simulink model "Multi_drones_deri_compare"  (R2021a)
settings: Solver=ode4  StartTime=0.0  StopTime=50  FixedStep=0.005  RelTol=1e-3
(part 3 of 7)

== system Multi_drones_deri_compare/Controller 6/Controller/Attitude controller ==
  states_i : Inport
  atti_ref : Inport  Port=2
  u_nom_a : Inport  Port=3
  Angle controller : MATLAB Function  TreatAsAtomicUnit=on
  Angle error : MATLAB Function  TreatAsAtomicUnit=on
  Angle sliding variable : MATLAB Function  TreatAsAtomicUnit=on
  Attitude loop observer : Subsystem
      settings: PortSchema="{\"entries\":[{\"content\":{\"sides\":[{\"content\":{\"connectorIds\":[\"In1\",\"In2\",\"In3\"]},\"type\":\"ConnectorPlacement.EquallySpacedRectSide\",\"uuid\":\"edf82c9f-eb15-4775-9311-d50d92fa47fd\"},{\"content\":{\"connectorIds\":[\"Out1\",\"Out2\"],\"side\":\"RIGHT\"},\"type\":\"ConnectorPlacement.EquallySpacedRectSide\",\"uuid\":\"b90416f6-8117-4ec7-8f9a-c5fae9711eab\"},{\"content\":{\"connectorIds\":[\"In4\"],\"side\":\"TOP\"},\"type\":\"ConnectorPlacement.EquallySpacedRectSide\",\"uuid\":\"e7e2e1a9-76d3-420a-917d-b73182cbe298\"}]},\"type\":\"ConnectorPlacement.EquallySpacedConnector\",\"uuid\":\"4fc8298e-c3da-4bdd-b1ba-c07bafbec956\"}],\"packageUris\":[\"http://schema.mathworks.com/mf0/Connector/R2020b\"],\"version\":\"1.0\"}"
  Scope : Scope
  Sliding mode differentiator : Subsystem
      settings: PortSchema="{\"entries\":[{\"content\":{\"sides\":[{\"content\":{\"connectorIds\":[\"In1\"]},\"type\":\"ConnectorPlacement.EquallySpacedRectSide\",\"uuid\":\"d0355641-aeac-4820-b7cd-f9621efbd127\"},{\"content\":{\"connectorIds\":[\"Out1\",\"Out2\"],\"side\":\"RIGHT\"},\"type\":\"ConnectorPlacement.EquallySpacedRectSide\",\"uuid\":\"185ec072-6206-4946-bebc-a6564ad10b6f\"},{\"content\":{\"connectorIds\":[\"Out3\"],\"side\":\"TOP\"},\"type\":\"ConnectorPlacement.EquallySpacedRectSide\",\"uuid\":\"43c1499b-0abd-4d60-8d0e-f99edfc99abb\"}]},\"type\":\"ConnectorPlacement.EquallySpacedConnector\",\"uuid\":\"7137f0d1-a693-433d-9f21-56f33280b1ef\"}],\"packageUris\":[\"http://schema.mathworks.com/mf0/Connector/R2020b\"],\"version\":\"1.0\"}"
  State selection : MATLAB Function  TreatAsAtomicUnit=on
  delta_v_a_6 : Scope
  delta_x_a_6 : Scope
  s_i_a_6 : Scope
  u_I_a : Outport
  w_hat_a : Outport  Port=2
  wires:
  Angle controller/1(u_i_a) -> Scope/1, u_I_a/1
  Angle sliding variable/1(s_i_a) -> s_i_a_6/1, Angle controller/2(s_i_a)
  atti_ref/1 -> Sliding mode differentiator/1(Reference)
  states_i/1 -> State selection/1(states_i), Attitude loop observer/1(states_i)
  State selection/1(x_i_a) -> Attitude loop observer/2(x_i_a), Angle error/1(x_i_a)
  State selection/2(v_i_a) -> Attitude loop observer/3(v_i_a), Angle error/2(v_i_a)
  Sliding mode differentiator/3(ang_d) -> Angle error/3(ang_d)
  Angle error/1(delta_x_a) -> delta_x_a_6/1, Angle sliding variable/1(delta_x_a), Angle controller/3(delta_x_a)
  Angle error/2(delta_v_a) -> delta_v_a_6/1, Angle controller/4(delta_v_a), Angle sliding variable/2(delta_v_a)
  Attitude loop observer/2(w_hat_a) -> Angle controller/1(w_hat_a)
  Sliding mode differentiator/2(ang_d_ddot) -> Angle controller/5(ang_d_ddot)
  u_nom_a/1 -> Attitude loop observer/4(u_nom_a)
  Sliding mode differentiator/1(ang_d_dot) -> Angle error/4(ang_d_dot)
  Attitude loop observer/1(w_hat_a_actual) -> w_hat_a/1

== system Multi_drones_deri_compare/Controller 6/Controller/Position controller1 ==
  states_i : Inport
  ref_x_p : Inport  Port=2
  u_nom_p : Inport  Port=3
  Constant : Constant  Value=[0;0;0]  VectorParams1D=off
  Error calculation : MATLAB Function  TreatAsAtomicUnit=on
  Position loop observer : Subsystem  mask{InitialCondition=[0;-1;0]}
      mask prompts: InitialCondition "Simulink:blkprm_prompts:IntegratorInitCond"
      settings: PortSchema="{\"entries\":[{\"content\":{\"sides\":[{\"content\":{\"connectorIds\":[\"In1\",\"In2\",\"In3\"]},\"type\":\"ConnectorPlacement.EquallySpacedRectSide\",\"uuid\":\"edf82c9f-eb15-4775-9311-d50d92fa47fd\"},{\"content\":{\"connectorIds\":[\"Out1\",\"Out2\"],\"side\":\"RIGHT\"},\"type\":\"ConnectorPlacement.EquallySpacedRectSide\",\"uuid\":\"b90416f6-8117-4ec7-8f9a-c5fae9711eab\"},{\"content\":{\"connectorIds\":[\"In4\"],\"side\":\"TOP\"},\"type\":\"ConnectorPlacement.EquallySpacedRectSide\",\"uuid\":\"e7e2e1a9-76d3-420a-917d-b73182cbe298\"}]},\"type\":\"ConnectorPlacement.EquallySpacedConnector\",\"uuid\":\"4fc8298e-c3da-4bdd-b1ba-c07bafbec956\"}],\"packageUris\":[\"http://schema.mathworks.com/mf0/Connector/R2020b\"],\"version\":\"1.0\"}"
      mask TypeOptions InitialCondition: x_int/InitialCondition
      mask DialogControl InitialCondition Prompt: Initial condition:
  Reference selection (Low) : MATLAB Function  TreatAsAtomicUnit=on
  State selection : MATLAB Function  TreatAsAtomicUnit=on
  Virtual position controller : MATLAB Function  TreatAsAtomicUnit=on
  delta_v_p_6 : Scope
  delta_x_p_6 : Scope
  s_i_p_6 : Scope
  u_i : Scope
  u_i_p : Outport
  w_hat_p : Outport  Port=2
  wires:
  states_i/1 -> Position loop observer/1(states_i), State selection/1(states_i)
  ref_x_p/1 -> Reference selection (Low)/1(ref_x_p)
  Reference selection (Low)/1(x_i_p_d) -> Error calculation/4(x_i_p_d)
  Reference selection (Low)/2(v_i_p_d) -> Error calculation/5(v_i_p_d)
  State selection/2(v_i_p) -> Position loop observer/3(v_i_p), Error calculation/2(v_i_p)
  State selection/1(x_i_p) -> Position loop observer/2(x_i_p), Error calculation/1(x_i_p)
  u_nom_p/1 -> Position loop observer/4(u_nom_p)
  Position loop observer/2(w_hat_p) -> Virtual position controller/1(w_hat_p)
  Reference selection (Low)/3(a_i_p_d) -> Virtual position controller/5(a_i_p_d)
  Constant/1 -> Error calculation/3(Phi_i)
  Error calculation/3(delta_v_p) -> delta_v_p_6/1, Virtual position controller/4(delta_v_p)
  Error calculation/2(delta_x_p) -> delta_x_p_6/1, Virtual position controller/3(delta_x_p)
  Error calculation/1(s_i_p) -> s_i_p_6/1, Virtual position controller/2(s_i_p)
  Virtual position controller/1(u_i_p) -> u_i_p/1, u_i/1
  Position loop observer/1(w_hat_p_actual) -> w_hat_p/1

== system Multi_drones_deri_compare/Controller 6/Controller/Reverse calculation ==
  psi_id : Inport
  u_ip : Inport  Port=2
  states_i : Inport  Port=3
  Reverse calculation : MATLAB Function  TreatAsAtomicUnit=on
  State selection : MATLAB Function  TreatAsAtomicUnit=on
  atti_ref : Outport
  T_i_d : Outport  Port=2
  wires:
  Reverse calculation/2(T_i_d) -> T_i_d/1
  Reverse calculation/1(atti_ref) -> atti_ref/1
  states_i/1 -> State selection/1(states_i)
  State selection/1(x_i_a) -> Reverse calculation/3(x_i_a)
  u_ip/1 -> Reverse calculation/2(u_i_p)
  psi_id/1 -> Reverse calculation/1(psi_i_d)

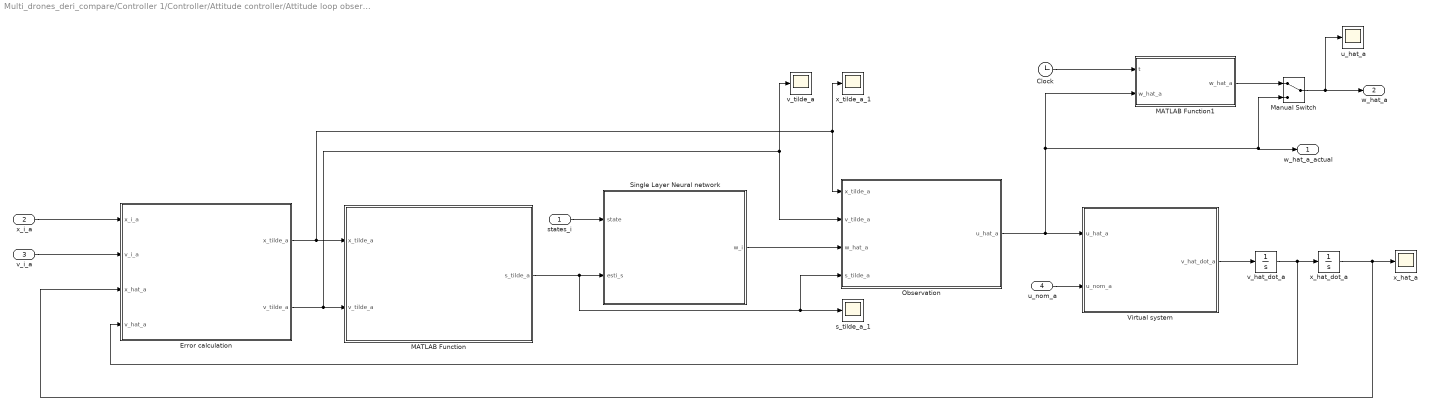
== system Multi_drones_deri_compare/Controller 1/Controller/Attitude controller/Attitude loop observer ==
  states_i : Inport
  x_i_a : Inport  Port=2
  v_i_a : Inport  Port=3
  u_nom_a : Inport  Port=4
  Clock : Clock
  Error calculation : MATLAB Function  TreatAsAtomicUnit=on
  MATLAB Function : MATLAB Function  TreatAsAtomicUnit=on
  MATLAB Function1 : MATLAB Function  TreatAsAtomicUnit=on
  Manual Switch : ManualSwitch
  Observation : MATLAB Function  TreatAsAtomicUnit=on
  Single Layer Neural network : Subsystem
  Virtual system : MATLAB Function  TreatAsAtomicUnit=on
  s_tilde_a_1 : Scope
  u_hat_a : Scope
  v_hat_dot_a : Integrator  InitialCondition=zeros(3,1)
  v_tilde_a : Scope
  x_hat_a : Scope
  x_hat_dot_a : Integrator  InitialCondition=zeros(3,1)
  x_tilde_a_1 : Scope
  w_hat_a_actual : Outport
  w_hat_a : Outport  Port=2
  wires:
  x_i_a/1 -> Error calculation/1(x_i_a)
  Error calculation/2(v_tilde_a) -> v_tilde_a/1, Observation/2(v_tilde_a), MATLAB Function/2(v_tilde_a)
  x_hat_dot_a/1 -> Error calculation/3(x_hat_a), x_hat_a/1
  v_hat_dot_a/1 -> Error calculation/4(v_hat_a), x_hat_dot_a/1
  MATLAB Function/1(s_tilde_a) -> Single Layer Neural network/2(esti_s), Observation/4(s_tilde_a), s_tilde_a_1/1
  Observation/1(u_hat_a) -> Manual Switch/2, w_hat_a_actual/1, MATLAB Function1/2("w_hat_a "), Virtual system/1(u_hat_a)
  u_nom_a/1 -> Virtual system/2(u_nom_a)
  v_i_a/1 -> Error calculation/2(v_i_a)
  Virtual system/1(v_hat_dot_a) -> v_hat_dot_a/1
  Error calculation/1(x_tilde_a) -> x_tilde_a_1/1, Observation/1(x_tilde_a), MATLAB Function/1(x_tilde_a)
  Single Layer Neural network/1(w_i) -> Observation/3(w_hat_a)
  states_i/1 -> Single Layer Neural network/1(state)
  Clock/1 -> MATLAB Function1/1(t)
  MATLAB Function1/1(w_hat_a) -> Manual Switch/1
  Manual Switch/1 -> u_hat_a/1, w_hat_a/1

== system Multi_drones_deri_compare/Controller 1/Controller/Attitude controller/Sliding mode differentiator ==
  note: Update initial state
  Reference : Inport
  Clock : Clock
  Constant : Constant  Value=[0;0;0]
  First-order derivative : Subsystem
  Integrator : Integrator  Commented=on  InitialCondition=[0;0;0;0;0;0;0;0;0;0;0;0]  ContinuousStateAttributes='speed'
  MATLAB Function : MATLAB Function  Commented=on  TreatAsAtomicUnit=on
  Manual Switch : ManualSwitch
  Second-order derivative : Subsystem
  a_d_a : Scope
  satu_atti_ref_ddot : Saturate  UpperLimit=0.1  LowerLimit=-0.1
  satu_atti_ref_dot : Saturate  UpperLimit=0.2  LowerLimit=-0.2
  sliding mode differentiator : MATLAB Function  Commented=on  TreatAsAtomicUnit=on
  v_d_a : Scope
  x_d_a : Scope
  ang_d_dot : Outport
  ang_d_ddot : Outport  Port=2
  ang_d : Outport  Port=3
  wires:
  sliding mode differentiator/1(z_dot) -> Integrator/1
  Reference/1 -> sliding mode differentiator/2(x_d), x_d_a/1, First-order derivative/1(ang_d), ang_d/1
  Integrator/1 -> MATLAB Function/1(z), sliding mode differentiator/1(z)
  satu_atti_ref_ddot/1 -> Manual Switch/1, a_d_a/1
  Second-order derivative/1(ang_d_ddot) -> satu_atti_ref_ddot/1
  Manual Switch/1 -> ang_d_ddot/1
  Constant/1 -> Manual Switch/2
  satu_atti_ref_dot/1 -> v_d_a/1, ang_d_dot/1
  Clock/1 -> Second-order derivative/2(t), First-order derivative/2(t)
  First-order derivative/1(ang_d_dot) -> satu_atti_ref_dot/1, Second-order derivative/1(ang_d_dot)

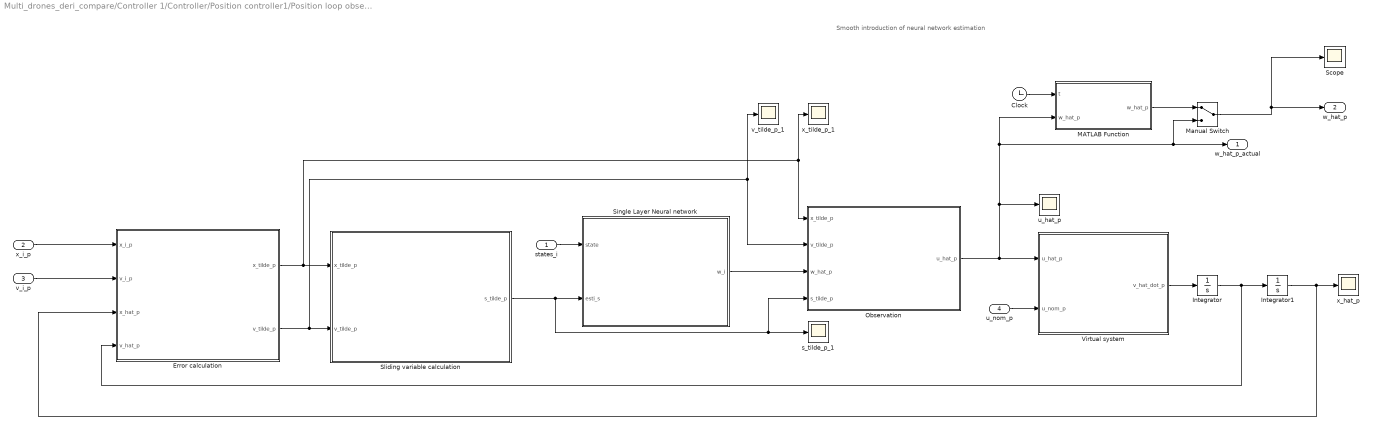
== system Multi_drones_deri_compare/Controller 1/Controller/Position controller1/Position loop observer ==
  note: Smooth introduction of neural network estimation
  states_i : Inport
  x_i_p : Inport  Port=2
  v_i_p : Inport  Port=3
  u_nom_p : Inport  Port=4
  Clock : Clock
  Error calculation : MATLAB Function  TreatAsAtomicUnit=on
  Integrator : Integrator  InitialCondition=[0;0;0]
  Integrator1 : Integrator  InitialCondition=InitialCondition
  MATLAB Function : MATLAB Function  TreatAsAtomicUnit=on
  Manual Switch : ManualSwitch
  Observation : MATLAB Function  TreatAsAtomicUnit=on
  Scope : Scope
  Single Layer Neural network : Subsystem
  Sliding variable calculation : MATLAB Function  TreatAsAtomicUnit=on
  Virtual system : MATLAB Function  TreatAsAtomicUnit=on
  s_tilde_p_1 : Scope
  u_hat_p : Scope
  v_tilde_p_1 : Scope
  x_hat_p : Scope
  x_tilde_p_1 : Scope
  w_hat_p_actual : Outport
  w_hat_p : Outport  Port=2
  wires:
  x_i_p/1 -> Error calculation/1(x_i_p)
  MATLAB Function/1(w_hat_p) -> Manual Switch/1
  Error calculation/2(v_tilde_p) -> v_tilde_p_1/1, Observation/2(v_tilde_p), Sliding variable calculation/2(v_tilde_p)
  Integrator1/1 -> Error calculation/3(x_hat_p), x_hat_p/1
  Integrator/1 -> Integrator1/1, Error calculation/4(v_hat_p)
  Sliding variable calculation/1(s_tilde_p) -> Single Layer Neural network/2(esti_s), Observation/4(s_tilde_p), s_tilde_p_1/1
  Observation/1(u_hat_p) -> w_hat_p_actual/1, Manual Switch/2, MATLAB Function/2("w_hat_p "), u_hat_p/1, Virtual system/1(u_hat_p)
  u_nom_p/1 -> Virtual system/2(u_nom_p)
  v_i_p/1 -> Error calculation/2(v_i_p)
  Virtual system/1(v_hat_dot_p) -> Integrator/1
  Error calculation/1(x_tilde_p) -> x_tilde_p_1/1, Observation/1(x_tilde_p), Sliding variable calculation/1(x_tilde_p)
  Single Layer Neural network/1(w_i) -> Observation/3(w_hat_p)
  states_i/1 -> Single Layer Neural network/1(state)
  Clock/1 -> MATLAB Function/1(t)
  Manual Switch/1 -> Scope/1, w_hat_p/1

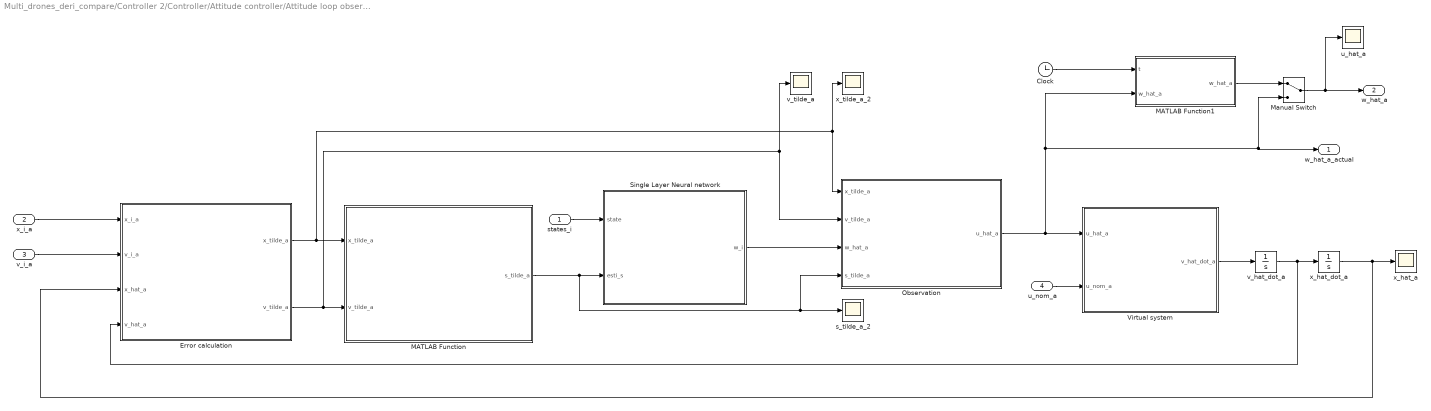
== system Multi_drones_deri_compare/Controller 2/Controller/Attitude controller/Attitude loop observer ==
  states_i : Inport
  x_i_a : Inport  Port=2
  v_i_a : Inport  Port=3
  u_nom_a : Inport  Port=4
  Clock : Clock
  Error calculation : MATLAB Function  TreatAsAtomicUnit=on
  MATLAB Function : MATLAB Function  TreatAsAtomicUnit=on
  MATLAB Function1 : MATLAB Function  TreatAsAtomicUnit=on
  Manual Switch : ManualSwitch
  Observation : MATLAB Function  TreatAsAtomicUnit=on
  Single Layer Neural network : Subsystem
  Virtual system : MATLAB Function  TreatAsAtomicUnit=on
  s_tilde_a_2 : Scope
  u_hat_a : Scope
  v_hat_dot_a : Integrator  InitialCondition=zeros(3,1)
  v_tilde_a : Scope
  x_hat_a : Scope
  x_hat_dot_a : Integrator  InitialCondition=zeros(3,1)
  x_tilde_a_2 : Scope
  w_hat_a_actual : Outport
  w_hat_a : Outport  Port=2
  wires:
  x_i_a/1 -> Error calculation/1(x_i_a)
  Error calculation/2(v_tilde_a) -> v_tilde_a/1, Observation/2(v_tilde_a), MATLAB Function/2(v_tilde_a)
  x_hat_dot_a/1 -> Error calculation/3(x_hat_a), x_hat_a/1
  v_hat_dot_a/1 -> Error calculation/4(v_hat_a), x_hat_dot_a/1
  MATLAB Function/1(s_tilde_a) -> Single Layer Neural network/2(esti_s), Observation/4(s_tilde_a), s_tilde_a_2/1
  Observation/1(u_hat_a) -> Manual Switch/2, w_hat_a_actual/1, MATLAB Function1/2("w_hat_a "), Virtual system/1(u_hat_a)
  u_nom_a/1 -> Virtual system/2(u_nom_a)
  v_i_a/1 -> Error calculation/2(v_i_a)
  Virtual system/1(v_hat_dot_a) -> v_hat_dot_a/1
  Error calculation/1(x_tilde_a) -> x_tilde_a_2/1, Observation/1(x_tilde_a), MATLAB Function/1(x_tilde_a)
  Single Layer Neural network/1(w_i) -> Observation/3(w_hat_a)
  states_i/1 -> Single Layer Neural network/1(state)
  Clock/1 -> MATLAB Function1/1(t)
  MATLAB Function1/1(w_hat_a) -> Manual Switch/1
  Manual Switch/1 -> u_hat_a/1, w_hat_a/1

== system Multi_drones_deri_compare/Controller 2/Controller/Attitude controller/Sliding mode differentiator ==
  note: Update initial state
  Reference : Inport
  Clock : Clock
  Constant : Constant  Value=[0;0;0]
  First-order derivative : Subsystem
  Integrator : Integrator  Commented=on  InitialCondition=[0;0;0;0;0;0;0;0;0;0;0;0]  ContinuousStateAttributes='speed'
  MATLAB Function : MATLAB Function  Commented=on  TreatAsAtomicUnit=on
  Manual Switch : ManualSwitch
  Second-order derivative : Subsystem
  a_d_a : Scope
  satu_atti_ref_ddot : Saturate  UpperLimit=0.2  LowerLimit=-0.2
  satu_atti_ref_dot : Saturate  UpperLimit=0.2  LowerLimit=-0.2
  sliding mode differentiator : MATLAB Function  Commented=on  TreatAsAtomicUnit=on
  v_d_a : Scope
  x_d_a : Scope
  ang_d_dot : Outport
  ang_d_ddot : Outport  Port=2
  ang_d : Outport  Port=3
  wires:
  sliding mode differentiator/1(z_dot) -> Integrator/1
  Reference/1 -> sliding mode differentiator/2(x_d), x_d_a/1, First-order derivative/1(ang_d), ang_d/1
  Integrator/1 -> MATLAB Function/1(z), sliding mode differentiator/1(z)
  satu_atti_ref_ddot/1 -> Manual Switch/1, a_d_a/1
  Second-order derivative/1(ang_d_ddot) -> satu_atti_ref_ddot/1
  Manual Switch/1 -> ang_d_ddot/1
  Constant/1 -> Manual Switch/2
  satu_atti_ref_dot/1 -> v_d_a/1, ang_d_dot/1
  Clock/1 -> Second-order derivative/2(t), First-order derivative/2(t)
  First-order derivative/1(ang_d_dot) -> satu_atti_ref_dot/1, Second-order derivative/1(ang_d_dot)

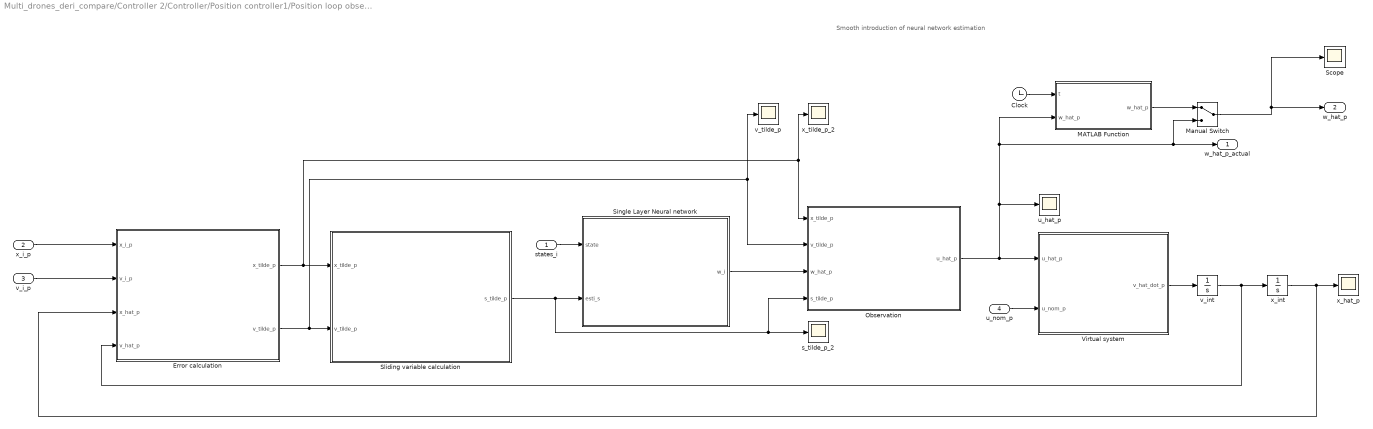
== system Multi_drones_deri_compare/Controller 2/Controller/Position controller1/Position loop observer ==
  note: Smooth introduction of neural network estimation
  states_i : Inport
  x_i_p : Inport  Port=2
  v_i_p : Inport  Port=3
  u_nom_p : Inport  Port=4
  Clock : Clock
  Error calculation : MATLAB Function  TreatAsAtomicUnit=on
  MATLAB Function : MATLAB Function  TreatAsAtomicUnit=on
  Manual Switch : ManualSwitch
  Observation : MATLAB Function  TreatAsAtomicUnit=on
  Scope : Scope
  Single Layer Neural network : Subsystem
  Sliding variable calculation : MATLAB Function  TreatAsAtomicUnit=on
  Virtual system : MATLAB Function  TreatAsAtomicUnit=on
  s_tilde_p_2 : Scope
  u_hat_p : Scope
  v_int : Integrator  InitialCondition=[0;0;0]
  v_tilde_p : Scope
  x_hat_p : Scope
  x_int : Integrator  InitialCondition=InitialCondition
  x_tilde_p_2 : Scope
  w_hat_p_actual : Outport
  w_hat_p : Outport  Port=2
  wires:
  x_i_p/1 -> Error calculation/1(x_i_p)
  MATLAB Function/1(w_hat_p) -> Manual Switch/1
  Error calculation/2(v_tilde_p) -> v_tilde_p/1, Observation/2(v_tilde_p), Sliding variable calculation/2(v_tilde_p)
  x_int/1 -> Error calculation/3(x_hat_p), x_hat_p/1
  v_int/1 -> x_int/1, Error calculation/4(v_hat_p)
  Sliding variable calculation/1(s_tilde_p) -> Single Layer Neural network/2(esti_s), Observation/4(s_tilde_p), s_tilde_p_2/1
  Observation/1(u_hat_p) -> w_hat_p_actual/1, Manual Switch/2, MATLAB Function/2("w_hat_p "), u_hat_p/1, Virtual system/1(u_hat_p)
  u_nom_p/1 -> Virtual system/2(u_nom_p)
  v_i_p/1 -> Error calculation/2(v_i_p)
  Virtual system/1(v_hat_dot_p) -> v_int/1
  Error calculation/1(x_tilde_p) -> x_tilde_p_2/1, Observation/1(x_tilde_p), Sliding variable calculation/1(x_tilde_p)
  Single Layer Neural network/1(w_i) -> Observation/3(w_hat_p)
  states_i/1 -> Single Layer Neural network/1(state)
  Clock/1 -> MATLAB Function/1(t)
  Manual Switch/1 -> Scope/1, w_hat_p/1

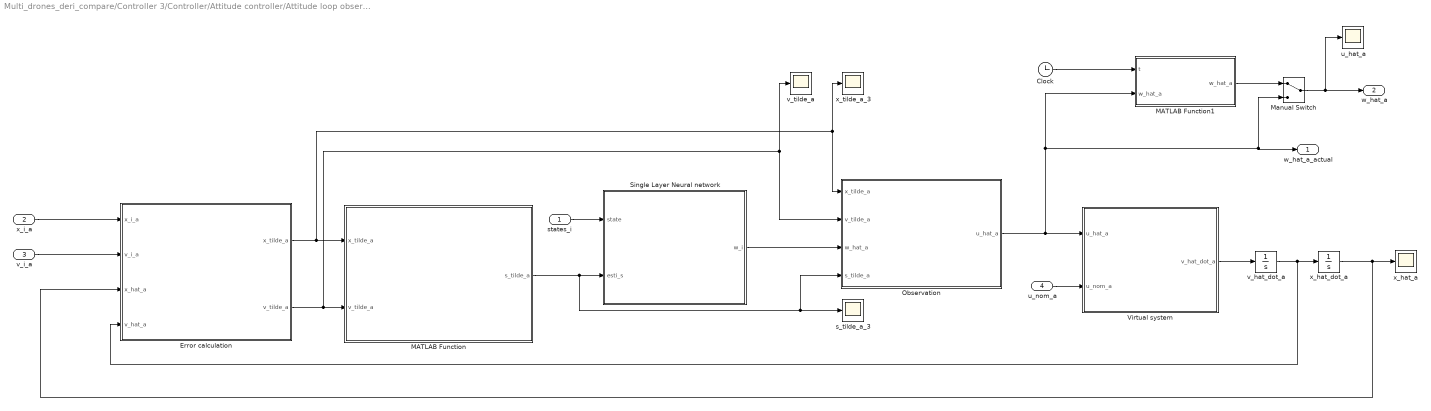
== system Multi_drones_deri_compare/Controller 3/Controller/Attitude controller/Attitude loop observer ==
  states_i : Inport
  x_i_a : Inport  Port=2
  v_i_a : Inport  Port=3
  u_nom_a : Inport  Port=4
  Clock : Clock
  Error calculation : MATLAB Function  TreatAsAtomicUnit=on
  MATLAB Function : MATLAB Function  TreatAsAtomicUnit=on
  MATLAB Function1 : MATLAB Function  TreatAsAtomicUnit=on
  Manual Switch : ManualSwitch
  Observation : MATLAB Function  TreatAsAtomicUnit=on
  Single Layer Neural network : Subsystem
  Virtual system : MATLAB Function  TreatAsAtomicUnit=on
  s_tilde_a_3 : Scope
  u_hat_a : Scope
  v_hat_dot_a : Integrator  InitialCondition=zeros(3,1)
  v_tilde_a : Scope
  x_hat_a : Scope
  x_hat_dot_a : Integrator  InitialCondition=zeros(3,1)
  x_tilde_a_3 : Scope
  w_hat_a_actual : Outport
  w_hat_a : Outport  Port=2
  wires:
  x_i_a/1 -> Error calculation/1(x_i_a)
  Error calculation/2(v_tilde_a) -> v_tilde_a/1, Observation/2(v_tilde_a), MATLAB Function/2(v_tilde_a)
  x_hat_dot_a/1 -> Error calculation/3(x_hat_a), x_hat_a/1
  v_hat_dot_a/1 -> Error calculation/4(v_hat_a), x_hat_dot_a/1
  MATLAB Function/1(s_tilde_a) -> Single Layer Neural network/2(esti_s), Observation/4(s_tilde_a), s_tilde_a_3/1
  Observation/1(u_hat_a) -> w_hat_a_actual/1, Manual Switch/2, MATLAB Function1/2("w_hat_a "), Virtual system/1(u_hat_a)
  u_nom_a/1 -> Virtual system/2(u_nom_a)
  v_i_a/1 -> Error calculation/2(v_i_a)
  Virtual system/1(v_hat_dot_a) -> v_hat_dot_a/1
  Error calculation/1(x_tilde_a) -> x_tilde_a_3/1, Observation/1(x_tilde_a), MATLAB Function/1(x_tilde_a)
  Single Layer Neural network/1(w_i) -> Observation/3(w_hat_a)
  states_i/1 -> Single Layer Neural network/1(state)
  Clock/1 -> MATLAB Function1/1(t)
  MATLAB Function1/1(w_hat_a) -> Manual Switch/1
  Manual Switch/1 -> u_hat_a/1, w_hat_a/1

== system Multi_drones_deri_compare/Controller 3/Controller/Attitude controller/Sliding mode differentiator ==
  note: Update initial state
  Reference : Inport
  Clock : Clock
  Constant : Constant  Value=[0;0;0]
  First-order derivative : Subsystem
  Integrator : Integrator  Commented=on  InitialCondition=[0;0;0;0;0;0;0;0;0;0;0;0]  ContinuousStateAttributes='speed'
  MATLAB Function : MATLAB Function  Commented=on  TreatAsAtomicUnit=on
  Manual Switch : ManualSwitch
  Second-order derivative : Subsystem
  a_d_a : Scope
  satu_atti_ref_ddot : Saturate  UpperLimit=0.2  LowerLimit=-0.2
  satu_atti_ref_dot : Saturate  UpperLimit=0.2  LowerLimit=-0.2
  sliding mode differentiator : MATLAB Function  Commented=on  TreatAsAtomicUnit=on
  v_d_a : Scope
  x_d_a : Scope
  ang_d_dot : Outport
  ang_d_ddot : Outport  Port=2
  ang_d : Outport  Port=3
  wires:
  sliding mode differentiator/1(z_dot) -> Integrator/1
  Reference/1 -> sliding mode differentiator/2(x_d), x_d_a/1, First-order derivative/1(ang_d), ang_d/1
  Integrator/1 -> MATLAB Function/1(z), sliding mode differentiator/1(z)
  satu_atti_ref_ddot/1 -> Manual Switch/1, a_d_a/1
  Second-order derivative/1(ang_d_ddot) -> satu_atti_ref_ddot/1
  Manual Switch/1 -> ang_d_ddot/1
  Constant/1 -> Manual Switch/2
  satu_atti_ref_dot/1 -> v_d_a/1, ang_d_dot/1
  Clock/1 -> Second-order derivative/2(t), First-order derivative/2(t)
  First-order derivative/1(ang_d_dot) -> satu_atti_ref_dot/1, Second-order derivative/1(ang_d_dot)

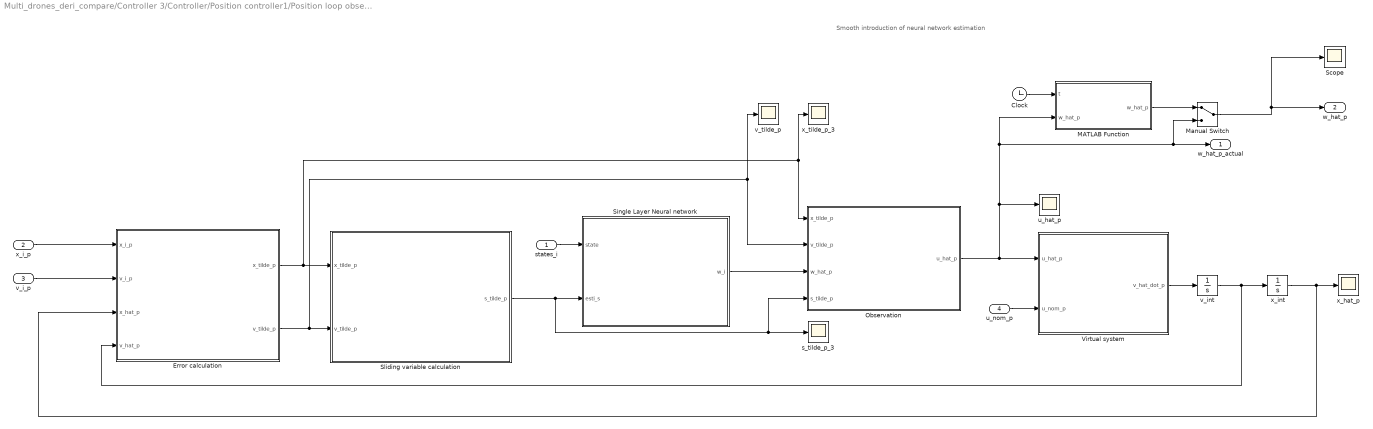
== system Multi_drones_deri_compare/Controller 3/Controller/Position controller1/Position loop observer ==
  note: Smooth introduction of neural network estimation
  states_i : Inport
  x_i_p : Inport  Port=2
  v_i_p : Inport  Port=3
  u_nom_p : Inport  Port=4
  Clock : Clock
  Error calculation : MATLAB Function  TreatAsAtomicUnit=on
  MATLAB Function : MATLAB Function  TreatAsAtomicUnit=on
  Manual Switch : ManualSwitch
  Observation : MATLAB Function  TreatAsAtomicUnit=on
  Scope : Scope
  Single Layer Neural network : Subsystem
  Sliding variable calculation : MATLAB Function  TreatAsAtomicUnit=on
  Virtual system : MATLAB Function  TreatAsAtomicUnit=on
  s_tilde_p_3 : Scope
  u_hat_p : Scope
  v_int : Integrator  InitialCondition=[0;0;0]
  v_tilde_p : Scope
  x_hat_p : Scope
  x_int : Integrator  InitialCondition=InitialCondition
  x_tilde_p_3 : Scope
  w_hat_p_actual : Outport
  w_hat_p : Outport  Port=2
  wires:
  x_i_p/1 -> Error calculation/1(x_i_p)
  MATLAB Function/1(w_hat_p) -> Manual Switch/1
  Error calculation/2(v_tilde_p) -> v_tilde_p/1, Observation/2(v_tilde_p), Sliding variable calculation/2(v_tilde_p)
  x_int/1 -> Error calculation/3(x_hat_p), x_hat_p/1
  v_int/1 -> x_int/1, Error calculation/4(v_hat_p)
  Sliding variable calculation/1(s_tilde_p) -> Single Layer Neural network/2(esti_s), Observation/4(s_tilde_p), s_tilde_p_3/1
  Observation/1(u_hat_p) -> w_hat_p_actual/1, Manual Switch/2, MATLAB Function/2("w_hat_p "), u_hat_p/1, Virtual system/1(u_hat_p)
  u_nom_p/1 -> Virtual system/2(u_nom_p)
  v_i_p/1 -> Error calculation/2(v_i_p)
  Virtual system/1(v_hat_dot_p) -> v_int/1
  Error calculation/1(x_tilde_p) -> x_tilde_p_3/1, Observation/1(x_tilde_p), Sliding variable calculation/1(x_tilde_p)
  Single Layer Neural network/1(w_i) -> Observation/3(w_hat_p)
  states_i/1 -> Single Layer Neural network/1(state)
  Clock/1 -> MATLAB Function/1(t)
  Manual Switch/1 -> Scope/1, w_hat_p/1

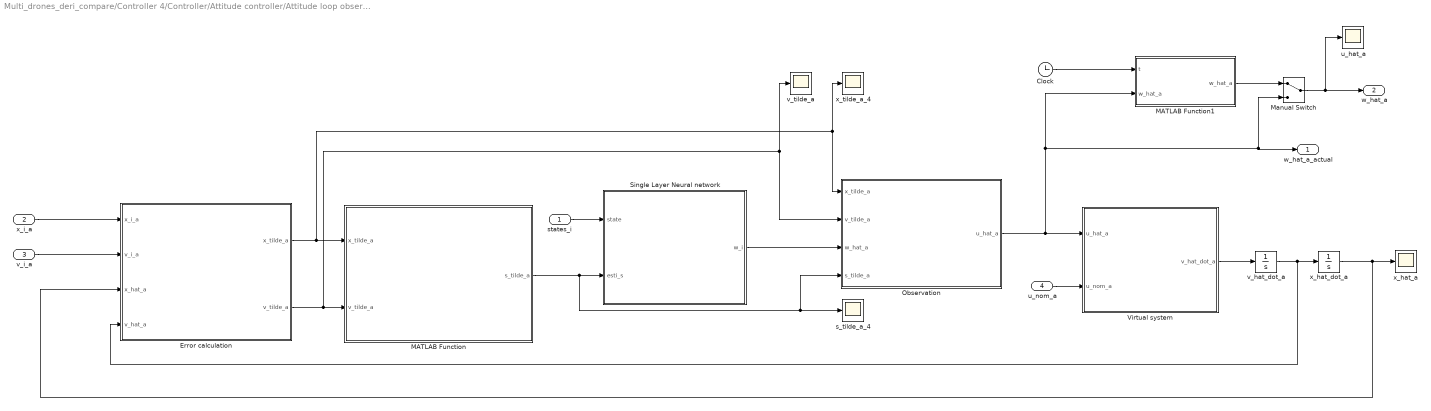
== system Multi_drones_deri_compare/Controller 4/Controller/Attitude controller/Attitude loop observer ==
  states_i : Inport
  x_i_a : Inport  Port=2
  v_i_a : Inport  Port=3
  u_nom_a : Inport  Port=4
  Clock : Clock
  Error calculation : MATLAB Function  TreatAsAtomicUnit=on
  MATLAB Function : MATLAB Function  TreatAsAtomicUnit=on
  MATLAB Function1 : MATLAB Function  TreatAsAtomicUnit=on
  Manual Switch : ManualSwitch
  Observation : MATLAB Function  TreatAsAtomicUnit=on
  Single Layer Neural network : Subsystem
  Virtual system : MATLAB Function  TreatAsAtomicUnit=on
  s_tilde_a_4 : Scope
  u_hat_a : Scope
  v_hat_dot_a : Integrator  InitialCondition=zeros(3,1)
  v_tilde_a : Scope
  x_hat_a : Scope
  x_hat_dot_a : Integrator  InitialCondition=zeros(3,1)
  x_tilde_a_4 : Scope
  w_hat_a_actual : Outport
  w_hat_a : Outport  Port=2
  wires:
  x_i_a/1 -> Error calculation/1(x_i_a)
  Error calculation/2(v_tilde_a) -> v_tilde_a/1, Observation/2(v_tilde_a), MATLAB Function/2(v_tilde_a)
  x_hat_dot_a/1 -> Error calculation/3(x_hat_a), x_hat_a/1
  v_hat_dot_a/1 -> Error calculation/4(v_hat_a), x_hat_dot_a/1
  MATLAB Function/1(s_tilde_a) -> Single Layer Neural network/2(esti_s), Observation/4(s_tilde_a), s_tilde_a_4/1
  Observation/1(u_hat_a) -> w_hat_a_actual/1, Manual Switch/2, MATLAB Function1/2("w_hat_a "), Virtual system/1(u_hat_a)
  u_nom_a/1 -> Virtual system/2(u_nom_a)
  v_i_a/1 -> Error calculation/2(v_i_a)
  Virtual system/1(v_hat_dot_a) -> v_hat_dot_a/1
  Error calculation/1(x_tilde_a) -> x_tilde_a_4/1, Observation/1(x_tilde_a), MATLAB Function/1(x_tilde_a)
  Single Layer Neural network/1(w_i) -> Observation/3(w_hat_a)
  states_i/1 -> Single Layer Neural network/1(state)
  Clock/1 -> MATLAB Function1/1(t)
  MATLAB Function1/1(w_hat_a) -> Manual Switch/1
  Manual Switch/1 -> u_hat_a/1, w_hat_a/1

== system Multi_drones_deri_compare/Controller 4/Controller/Attitude controller/Sliding mode differentiator ==
  note: Update initial state
  Reference : Inport
  Clock : Clock
  Constant : Constant  Value=[0;0;0]
  First-order derivative : Subsystem
  Integrator : Integrator  Commented=on  InitialCondition=[0;0;0;0;0;0;0;0;0;0;0;0]  ContinuousStateAttributes='speed'
  MATLAB Function : MATLAB Function  Commented=on  TreatAsAtomicUnit=on
  Manual Switch : ManualSwitch
  Second-order derivative : Subsystem
  a_d_a : Scope
  satu_atti_ref_ddot : Saturate  UpperLimit=0.2  LowerLimit=-0.2
  satu_atti_ref_dot : Saturate  UpperLimit=0.2  LowerLimit=-0.2
  sliding mode differentiator : MATLAB Function  Commented=on  TreatAsAtomicUnit=on
  v_d_a : Scope
  x_d_a : Scope
  ang_d_dot : Outport
  ang_d_ddot : Outport  Port=2
  ang_d : Outport  Port=3
  wires:
  sliding mode differentiator/1(z_dot) -> Integrator/1
  Reference/1 -> sliding mode differentiator/2(x_d), x_d_a/1, First-order derivative/1(ang_d), ang_d/1
  Integrator/1 -> MATLAB Function/1(z), sliding mode differentiator/1(z)
  satu_atti_ref_ddot/1 -> Manual Switch/1, a_d_a/1
  Second-order derivative/1(ang_d_ddot) -> satu_atti_ref_ddot/1
  Manual Switch/1 -> ang_d_ddot/1
  Constant/1 -> Manual Switch/2
  satu_atti_ref_dot/1 -> v_d_a/1, ang_d_dot/1
  Clock/1 -> Second-order derivative/2(t), First-order derivative/2(t)
  First-order derivative/1(ang_d_dot) -> satu_atti_ref_dot/1, Second-order derivative/1(ang_d_dot)

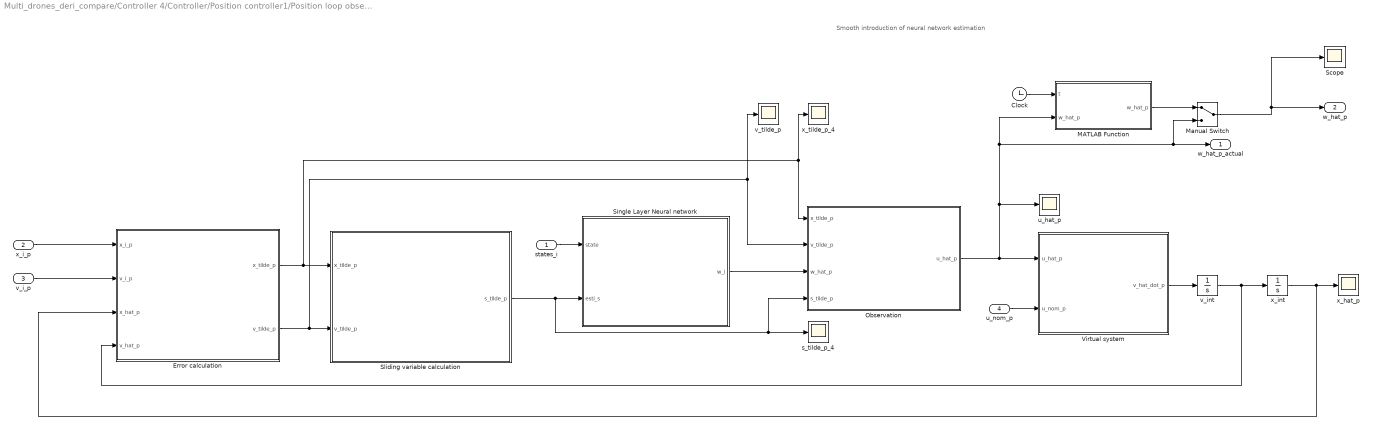
== system Multi_drones_deri_compare/Controller 4/Controller/Position controller1/Position loop observer ==
  note: Smooth introduction of neural network estimation
  states_i : Inport
  x_i_p : Inport  Port=2
  v_i_p : Inport  Port=3
  u_nom_p : Inport  Port=4
  Clock : Clock
  Error calculation : MATLAB Function  TreatAsAtomicUnit=on
  MATLAB Function : MATLAB Function  TreatAsAtomicUnit=on
  Manual Switch : ManualSwitch
  Observation : MATLAB Function  TreatAsAtomicUnit=on
  Scope : Scope
  Single Layer Neural network : Subsystem
  Sliding variable calculation : MATLAB Function  TreatAsAtomicUnit=on
  Virtual system : MATLAB Function  TreatAsAtomicUnit=on
  s_tilde_p_4 : Scope
  u_hat_p : Scope
  v_int : Integrator  InitialCondition=[0;0;0]
  v_tilde_p : Scope
  x_hat_p : Scope
  x_int : Integrator  InitialCondition=InitialCondition
  x_tilde_p_4 : Scope
  w_hat_p_actual : Outport
  w_hat_p : Outport  Port=2
  wires:
  x_i_p/1 -> Error calculation/1(x_i_p)
  MATLAB Function/1(w_hat_p) -> Manual Switch/1
  Error calculation/2(v_tilde_p) -> v_tilde_p/1, Observation/2(v_tilde_p), Sliding variable calculation/2(v_tilde_p)
  x_int/1 -> Error calculation/3(x_hat_p), x_hat_p/1
  v_int/1 -> x_int/1, Error calculation/4(v_hat_p)
  Sliding variable calculation/1(s_tilde_p) -> Single Layer Neural network/2(esti_s), Observation/4(s_tilde_p), s_tilde_p_4/1
  Observation/1(u_hat_p) -> w_hat_p_actual/1, Manual Switch/2, MATLAB Function/2("w_hat_p "), u_hat_p/1, Virtual system/1(u_hat_p)
  u_nom_p/1 -> Virtual system/2(u_nom_p)
  v_i_p/1 -> Error calculation/2(v_i_p)
  Virtual system/1(v_hat_dot_p) -> v_int/1
  Error calculation/1(x_tilde_p) -> x_tilde_p_4/1, Observation/1(x_tilde_p), Sliding variable calculation/1(x_tilde_p)
  Single Layer Neural network/1(w_i) -> Observation/3(w_hat_p)
  states_i/1 -> Single Layer Neural network/1(state)
  Clock/1 -> MATLAB Function/1(t)
  Manual Switch/1 -> Scope/1, w_hat_p/1

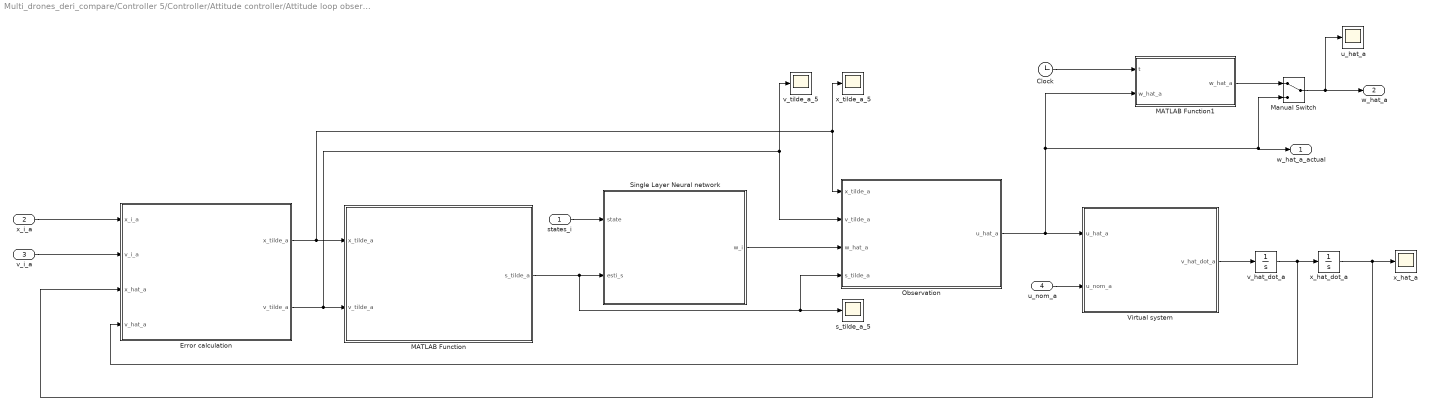
== system Multi_drones_deri_compare/Controller 5/Controller/Attitude controller/Attitude loop observer ==
  states_i : Inport
  x_i_a : Inport  Port=2
  v_i_a : Inport  Port=3
  u_nom_a : Inport  Port=4
  Clock : Clock
  Error calculation : MATLAB Function  TreatAsAtomicUnit=on
  MATLAB Function : MATLAB Function  TreatAsAtomicUnit=on
  MATLAB Function1 : MATLAB Function  TreatAsAtomicUnit=on
  Manual Switch : ManualSwitch
  Observation : MATLAB Function  TreatAsAtomicUnit=on
  Single Layer Neural network : Subsystem
  Virtual system : MATLAB Function  TreatAsAtomicUnit=on
  s_tilde_a_5 : Scope
  u_hat_a : Scope
  v_hat_dot_a : Integrator  InitialCondition=zeros(3,1)
  v_tilde_a_5 : Scope
  x_hat_a : Scope
  x_hat_dot_a : Integrator  InitialCondition=zeros(3,1)
  x_tilde_a_5 : Scope
  w_hat_a_actual : Outport
  w_hat_a : Outport  Port=2
  wires:
  x_i_a/1 -> Error calculation/1(x_i_a)
  Error calculation/2(v_tilde_a) -> v_tilde_a_5/1, Observation/2(v_tilde_a), MATLAB Function/2(v_tilde_a)
  x_hat_dot_a/1 -> Error calculation/3(x_hat_a), x_hat_a/1
  v_hat_dot_a/1 -> Error calculation/4(v_hat_a), x_hat_dot_a/1
  MATLAB Function/1(s_tilde_a) -> Single Layer Neural network/2(esti_s), Observation/4(s_tilde_a), s_tilde_a_5/1
  Observation/1(u_hat_a) -> Manual Switch/2, w_hat_a_actual/1, MATLAB Function1/2("w_hat_a "), Virtual system/1(u_hat_a)
  u_nom_a/1 -> Virtual system/2(u_nom_a)
  v_i_a/1 -> Error calculation/2(v_i_a)
  Virtual system/1(v_hat_dot_a) -> v_hat_dot_a/1
  Error calculation/1(x_tilde_a) -> x_tilde_a_5/1, Observation/1(x_tilde_a), MATLAB Function/1(x_tilde_a)
  Single Layer Neural network/1(w_i) -> Observation/3(w_hat_a)
  states_i/1 -> Single Layer Neural network/1(state)
  Clock/1 -> MATLAB Function1/1(t)
  MATLAB Function1/1(w_hat_a) -> Manual Switch/1
  Manual Switch/1 -> u_hat_a/1, w_hat_a/1

== system Multi_drones_deri_compare/Controller 5/Controller/Attitude controller/Sliding mode differentiator ==
  note: Update initial state
  Reference : Inport
  Clock : Clock
  Constant : Constant  Value=[0;0;0]
  First-order derivative : Subsystem
  Integrator : Integrator  Commented=on  InitialCondition=[0;0;0;0;0;0;0;0;0;0;0;0]  ContinuousStateAttributes='speed'
  MATLAB Function : MATLAB Function  Commented=on  TreatAsAtomicUnit=on
  Manual Switch : ManualSwitch
  Second-order derivative : Subsystem
  a_d_a : Scope
  satu_atti_ref_ddot : Saturate  UpperLimit=0.2  LowerLimit=-0.2
  satu_atti_ref_dot : Saturate  UpperLimit=0.2  LowerLimit=-0.2
  sliding mode differentiator : MATLAB Function  Commented=on  TreatAsAtomicUnit=on
  v_d_a : Scope
  x_d_a : Scope
  ang_d_dot : Outport
  ang_d_ddot : Outport  Port=2
  ang_d : Outport  Port=3
  wires:
  sliding mode differentiator/1(z_dot) -> Integrator/1
  Reference/1 -> sliding mode differentiator/2(x_d), x_d_a/1, First-order derivative/1(ang_d), ang_d/1
  Integrator/1 -> MATLAB Function/1(z), sliding mode differentiator/1(z)
  satu_atti_ref_ddot/1 -> Manual Switch/1, a_d_a/1
  Second-order derivative/1(ang_d_ddot) -> satu_atti_ref_ddot/1
  Manual Switch/1 -> ang_d_ddot/1
  Constant/1 -> Manual Switch/2
  satu_atti_ref_dot/1 -> v_d_a/1, ang_d_dot/1
  Clock/1 -> Second-order derivative/2(t), First-order derivative/2(t)
  First-order derivative/1(ang_d_dot) -> satu_atti_ref_dot/1, Second-order derivative/1(ang_d_dot)

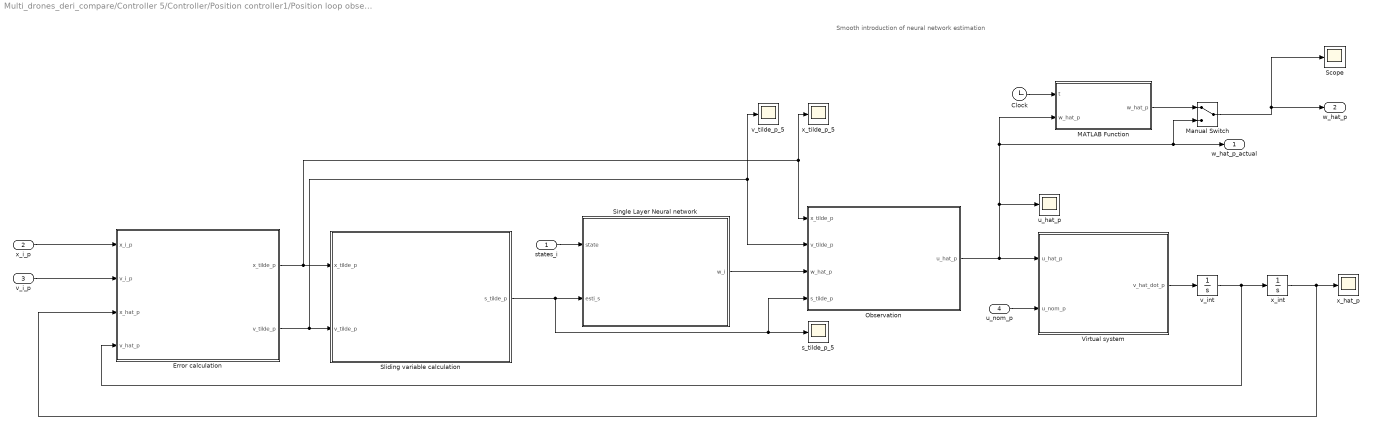
== system Multi_drones_deri_compare/Controller 5/Controller/Position controller1/Position loop observer ==
  note: Smooth introduction of neural network estimation
  states_i : Inport
  x_i_p : Inport  Port=2
  v_i_p : Inport  Port=3
  u_nom_p : Inport  Port=4
  Clock : Clock
  Error calculation : MATLAB Function  TreatAsAtomicUnit=on
  MATLAB Function : MATLAB Function  TreatAsAtomicUnit=on
  Manual Switch : ManualSwitch
  Observation : MATLAB Function  TreatAsAtomicUnit=on
  Scope : Scope
  Single Layer Neural network : Subsystem
  Sliding variable calculation : MATLAB Function  TreatAsAtomicUnit=on
  Virtual system : MATLAB Function  TreatAsAtomicUnit=on
  s_tilde_p_5 : Scope
  u_hat_p : Scope
  v_int : Integrator  InitialCondition=[0;0;0]
  v_tilde_p_5 : Scope
  x_hat_p : Scope
  x_int : Integrator  InitialCondition=InitialCondition
  x_tilde_p_5 : Scope
  w_hat_p_actual : Outport
  w_hat_p : Outport  Port=2
  wires:
  x_i_p/1 -> Error calculation/1(x_i_p)
  MATLAB Function/1(w_hat_p) -> Manual Switch/1
  Error calculation/2(v_tilde_p) -> v_tilde_p_5/1, Observation/2(v_tilde_p), Sliding variable calculation/2(v_tilde_p)
  x_int/1 -> Error calculation/3(x_hat_p), x_hat_p/1
  v_int/1 -> x_int/1, Error calculation/4(v_hat_p)
  Sliding variable calculation/1(s_tilde_p) -> Single Layer Neural network/2(esti_s), Observation/4(s_tilde_p), s_tilde_p_5/1
  Observation/1(u_hat_p) -> w_hat_p_actual/1, Manual Switch/2, MATLAB Function/2("w_hat_p "), u_hat_p/1, Virtual system/1(u_hat_p)
  u_nom_p/1 -> Virtual system/2(u_nom_p)
  v_i_p/1 -> Error calculation/2(v_i_p)
  Virtual system/1(v_hat_dot_p) -> v_int/1
  Error calculation/1(x_tilde_p) -> x_tilde_p_5/1, Observation/1(x_tilde_p), Sliding variable calculation/1(x_tilde_p)
  Single Layer Neural network/1(w_i) -> Observation/3(w_hat_p)
  states_i/1 -> Single Layer Neural network/1(state)
  Clock/1 -> MATLAB Function/1(t)
  Manual Switch/1 -> Scope/1, w_hat_p/1

== system Multi_drones_deri_compare/Controller 6/Controller/Attitude controller/Attitude loop observer ==
  states_i : Inport
  x_i_a : Inport  Port=2
  v_i_a : Inport  Port=3
  u_nom_a : Inport  Port=4
  Clock : Clock
  Error calculation : MATLAB Function  TreatAsAtomicUnit=on
  MATLAB Function : MATLAB Function  TreatAsAtomicUnit=on
  MATLAB Function1 : MATLAB Function  TreatAsAtomicUnit=on
  Manual Switch : ManualSwitch
  Observation : MATLAB Function  TreatAsAtomicUnit=on
  Single Layer Neural network : Subsystem
  Virtual system : MATLAB Function  TreatAsAtomicUnit=on
  s_tilde_a_6 : Scope
  u_hat_a : Scope
  v_hat_dot_a : Integrator  InitialCondition=zeros(3,1)
  v_tilde_a_6 : Scope
  x_hat_a : Scope
  x_hat_dot_a : Integrator  InitialCondition=zeros(3,1)
  x_tilde_a_6 : Scope
  w_hat_a_actual : Outport
  w_hat_a : Outport  Port=2
  wires:
  x_i_a/1 -> Error calculation/1(x_i_a)
  Error calculation/2(v_tilde_a) -> v_tilde_a_6/1, Observation/2(v_tilde_a), MATLAB Function/2(v_tilde_a)
  x_hat_dot_a/1 -> Error calculation/3(x_hat_a), x_hat_a/1
  v_hat_dot_a/1 -> Error calculation/4(v_hat_a), x_hat_dot_a/1
  MATLAB Function/1(s_tilde_a) -> Single Layer Neural network/2(esti_s), Observation/4(s_tilde_a), s_tilde_a_6/1
  Observation/1(u_hat_a) -> Manual Switch/2, w_hat_a_actual/1, MATLAB Function1/2("w_hat_a "), Virtual system/1(u_hat_a)
  u_nom_a/1 -> Virtual system/2(u_nom_a)
  v_i_a/1 -> Error calculation/2(v_i_a)
  Virtual system/1(v_hat_dot_a) -> v_hat_dot_a/1
  Error calculation/1(x_tilde_a) -> x_tilde_a_6/1, Observation/1(x_tilde_a), MATLAB Function/1(x_tilde_a)
  Single Layer Neural network/1(w_i) -> Observation/3(w_hat_a)
  states_i/1 -> Single Layer Neural network/1(state)
  Clock/1 -> MATLAB Function1/1(t)
  MATLAB Function1/1(w_hat_a) -> Manual Switch/1
  Manual Switch/1 -> u_hat_a/1, w_hat_a/1

== system Multi_drones_deri_compare/Controller 6/Controller/Attitude controller/Sliding mode differentiator ==
  note: Update initial state
  Reference : Inport
  Clock : Clock
  Constant : Constant  Value=[0;0;0]
  First-order derivative : Subsystem
  Integrator : Integrator  Commented=on  InitialCondition=[0;0;0;0;0;0;0;0;0;0;0;0]  ContinuousStateAttributes='speed'
  MATLAB Function : MATLAB Function  Commented=on  TreatAsAtomicUnit=on
  Manual Switch : ManualSwitch
  Second-order derivative : Subsystem
  a_d_a : Scope
  satu_atti_ref_ddot : Saturate  UpperLimit=0.2  LowerLimit=-0.2
  satu_atti_ref_dot : Saturate  UpperLimit=0.2  LowerLimit=-0.2
  sliding mode differentiator : MATLAB Function  Commented=on  TreatAsAtomicUnit=on
  v_d_a : Scope
  x_d_a : Scope
  ang_d_dot : Outport
  ang_d_ddot : Outport  Port=2
  ang_d : Outport  Port=3
  wires:
  sliding mode differentiator/1(z_dot) -> Integrator/1
  Reference/1 -> sliding mode differentiator/2(x_d), x_d_a/1, First-order derivative/1(ang_d), ang_d/1
  Integrator/1 -> MATLAB Function/1(z), sliding mode differentiator/1(z)
  satu_atti_ref_ddot/1 -> Manual Switch/1, a_d_a/1
  Second-order derivative/1(ang_d_ddot) -> satu_atti_ref_ddot/1
  Manual Switch/1 -> ang_d_ddot/1
  Constant/1 -> Manual Switch/2
  satu_atti_ref_dot/1 -> v_d_a/1, ang_d_dot/1
  Clock/1 -> Second-order derivative/2(t), First-order derivative/2(t)
  First-order derivative/1(ang_d_dot) -> satu_atti_ref_dot/1, Second-order derivative/1(ang_d_dot)

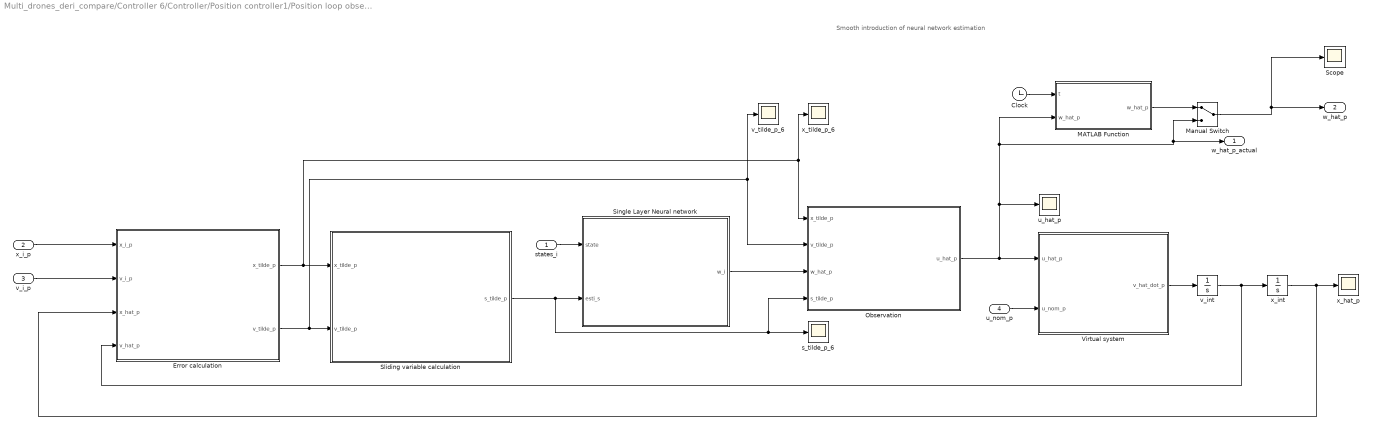
== system Multi_drones_deri_compare/Controller 6/Controller/Position controller1/Position loop observer ==
  note: Smooth introduction of neural network estimation
  states_i : Inport
  x_i_p : Inport  Port=2
  v_i_p : Inport  Port=3
  u_nom_p : Inport  Port=4
  Clock : Clock
  Error calculation : MATLAB Function  TreatAsAtomicUnit=on
  MATLAB Function : MATLAB Function  TreatAsAtomicUnit=on
  Manual Switch : ManualSwitch
  Observation : MATLAB Function  TreatAsAtomicUnit=on
  Scope : Scope
  Single Layer Neural network : Subsystem
  Sliding variable calculation : MATLAB Function  TreatAsAtomicUnit=on
  Virtual system : MATLAB Function  TreatAsAtomicUnit=on
  s_tilde_p_6 : Scope
  u_hat_p : Scope
  v_int : Integrator  InitialCondition=[0;0;0]
  v_tilde_p_6 : Scope
  x_hat_p : Scope
  x_int : Integrator  InitialCondition=InitialCondition
  x_tilde_p_6 : Scope
  w_hat_p_actual : Outport
  w_hat_p : Outport  Port=2
  wires:
  x_i_p/1 -> Error calculation/1(x_i_p)
  MATLAB Function/1(w_hat_p) -> Manual Switch/1
  Error calculation/2(v_tilde_p) -> v_tilde_p_6/1, Observation/2(v_tilde_p), Sliding variable calculation/2(v_tilde_p)
  x_int/1 -> Error calculation/3(x_hat_p), x_hat_p/1
  v_int/1 -> x_int/1, Error calculation/4(v_hat_p)
  Sliding variable calculation/1(s_tilde_p) -> Single Layer Neural network/2(esti_s), Observation/4(s_tilde_p), s_tilde_p_6/1
  Observation/1(u_hat_p) -> w_hat_p_actual/1, Manual Switch/2, MATLAB Function/2("w_hat_p "), u_hat_p/1, Virtual system/1(u_hat_p)
  u_nom_p/1 -> Virtual system/2(u_nom_p)
  v_i_p/1 -> Error calculation/2(v_i_p)
  Virtual system/1(v_hat_dot_p) -> v_int/1
  Error calculation/1(x_tilde_p) -> x_tilde_p_6/1, Observation/1(x_tilde_p), Sliding variable calculation/1(x_tilde_p)
  Single Layer Neural network/1(w_i) -> Observation/3(w_hat_p)
  states_i/1 -> Single Layer Neural network/1(state)
  Clock/1 -> MATLAB Function/1(t)
  Manual Switch/1 -> Scope/1, w_hat_p/1

== system Multi_drones_deri_compare/Controller 1/Controller/Attitude controller/Attitude loop observer/Single Layer Neural network ==
  state : Inport
  esti_s : Inport  Port=2
  Neural network output : MATLAB Function  TreatAsAtomicUnit=on
  Update of neural weight : MATLAB Function  TreatAsAtomicUnit=on
  Weight initialisation : MATLAB Function  TreatAsAtomicUnit=on
  Weight update : Integrator  InitialConditionSource=external
  w_i : Outport
  wires:
  Update of neural weight/1(W_dot) -> Weight update/1
  esti_s/1 -> Update of neural weight/2(esti_s)
  state/1 -> Update of neural weight/1(phi_net), Neural network output/1(phi_net)
  Neural network output/1(w_i) -> w_i/1
  Weight initialisation/1(W_0) -> Weight update/2
  Weight update/1 -> Update of neural weight/3(W), Neural network output/2(W)

== system Multi_drones_deri_compare/Controller 1/Controller/Attitude controller/Sliding mode differentiator/First-order derivative ==
  ang_d : Inport
  t : Inport  Port=2
  First derivative : MATLAB Function  TreatAsAtomicUnit=on
  Memory : Memory  InitialCondition=[0;0;0]
  Memory1 : Memory
  Memory2 : Memory  InitialCondition=[0;0;0]
  ang_d_dot : Outport
  wires:
  ang_d/1 -> First derivative/1(ang_d)
  First derivative/1(ang_d_dot) -> Memory2/1
  t/1 -> First derivative/2(t)
  First derivative/3(loop_num) -> Memory1/1
  Memory1/1 -> First derivative/5("loop_num ")
  First derivative/2(ang_d_prev) -> Memory/1
  Memory/1 -> First derivative/3("ang_d_prev ")
  Memory2/1 -> First derivative/4("ang_d_dot "), ang_d_dot/1

== system Multi_drones_deri_compare/Controller 1/Controller/Attitude controller/Sliding mode differentiator/Second-order derivative ==
  ang_d_dot : Inport
  t : Inport  Port=2
  First derivative : MATLAB Function  TreatAsAtomicUnit=on
  Memory : Memory  InitialCondition=[0;0;0]
  Memory1 : Memory
  Memory2 : Memory  InitialCondition=[0;0;0]
  ang_d_ddot : Outport
  wires:
  ang_d_dot/1 -> First derivative/1(ang_d_dot)
  First derivative/1(ang_d_ddot) -> Memory2/1
  t/1 -> First derivative/2(t)
  First derivative/3(loop_num) -> Memory1/1
  Memory1/1 -> First derivative/5("loop_num ")
  First derivative/2(ang_d_dot_prev) -> Memory/1
  Memory/1 -> First derivative/3("ang_d_dot_prev ")
  Memory2/1 -> First derivative/4("ang_d_ddot "), ang_d_ddot/1

== system Multi_drones_deri_compare/Controller 1/Controller/Position controller1/Position loop observer/Single Layer Neural network ==
  state : Inport
  esti_s : Inport  Port=2
  Neural network output : MATLAB Function  TreatAsAtomicUnit=on
  Update of neural weight : MATLAB Function  TreatAsAtomicUnit=on
  Weight initialisation : MATLAB Function  TreatAsAtomicUnit=on
  Weight update : Integrator  InitialConditionSource=external
  w_i : Outport
  wires:
  Update of neural weight/1(W_dot) -> Weight update/1
  esti_s/1 -> Update of neural weight/2(esti_s)
  state/1 -> Update of neural weight/1(phi_net), Neural network output/1(phi_net)
  Neural network output/1(w_i) -> w_i/1
  Weight initialisation/1(W_0) -> Weight update/2
  Weight update/1 -> Update of neural weight/3(W), Neural network output/2(W)

== system Multi_drones_deri_compare/Controller 2/Controller/Attitude controller/Attitude loop observer/Single Layer Neural network ==
  state : Inport
  esti_s : Inport  Port=2
  Neural network output : MATLAB Function  TreatAsAtomicUnit=on
  Update of neural weight : MATLAB Function  TreatAsAtomicUnit=on
  Weight initialisation : MATLAB Function  TreatAsAtomicUnit=on
  Weight update : Integrator  InitialConditionSource=external
  w_i : Outport
  wires:
  Update of neural weight/1(W_dot) -> Weight update/1
  esti_s/1 -> Update of neural weight/2(esti_s)
  state/1 -> Update of neural weight/1(phi_net), Neural network output/1(phi_net)
  Neural network output/1(w_i) -> w_i/1
  Weight initialisation/1(W_0) -> Weight update/2
  Weight update/1 -> Update of neural weight/3(W), Neural network output/2(W)

== system Multi_drones_deri_compare/Controller 2/Controller/Attitude controller/Sliding mode differentiator/First-order derivative ==
  ang_d : Inport
  t : Inport  Port=2
  First derivative : MATLAB Function  TreatAsAtomicUnit=on
  Memory : Memory  InitialCondition=[0;0;0]
  Memory1 : Memory
  Memory2 : Memory  InitialCondition=[0;0;0]
  ang_d_dot : Outport
  wires:
  ang_d/1 -> First derivative/1(ang_d)
  First derivative/1(ang_d_dot) -> Memory2/1
  t/1 -> First derivative/2(t)
  First derivative/3(loop_num) -> Memory1/1
  Memory1/1 -> First derivative/5("loop_num ")
  First derivative/2(ang_d_prev) -> Memory/1
  Memory/1 -> First derivative/3("ang_d_prev ")
  Memory2/1 -> First derivative/4("ang_d_dot "), ang_d_dot/1

== system Multi_drones_deri_compare/Controller 2/Controller/Attitude controller/Sliding mode differentiator/Second-order derivative ==
  ang_d_dot : Inport
  t : Inport  Port=2
  First derivative : MATLAB Function  TreatAsAtomicUnit=on
  Memory : Memory  InitialCondition=[0;0;0]
  Memory1 : Memory
  Memory2 : Memory  InitialCondition=[0;0;0]
  ang_d_ddot : Outport
  wires:
  ang_d_dot/1 -> First derivative/1(ang_d_dot)
  First derivative/1(ang_d_ddot) -> Memory2/1
  t/1 -> First derivative/2(t)
  First derivative/3(loop_num) -> Memory1/1
  Memory1/1 -> First derivative/5("loop_num ")
  First derivative/2(ang_d_dot_prev) -> Memory/1
  Memory/1 -> First derivative/3("ang_d_dot_prev ")
  Memory2/1 -> First derivative/4("ang_d_ddot "), ang_d_ddot/1

== system Multi_drones_deri_compare/Controller 2/Controller/Position controller1/Position loop observer/Single Layer Neural network ==
  state : Inport
  esti_s : Inport  Port=2
  Neural network output : MATLAB Function  TreatAsAtomicUnit=on
  Update of neural weight : MATLAB Function  TreatAsAtomicUnit=on
  Weight initialisation : MATLAB Function  TreatAsAtomicUnit=on
  Weight update : Integrator  InitialConditionSource=external
  w_i : Outport
  wires:
  Update of neural weight/1(W_dot) -> Weight update/1
  esti_s/1 -> Update of neural weight/2(esti_s)
  state/1 -> Update of neural weight/1(phi_net), Neural network output/1(phi_net)
  Neural network output/1(w_i) -> w_i/1
  Weight initialisation/1(W_0) -> Weight update/2
  Weight update/1 -> Update of neural weight/3(W), Neural network output/2(W)

== system Multi_drones_deri_compare/Controller 3/Controller/Attitude controller/Attitude loop observer/Single Layer Neural network ==
  state : Inport
  esti_s : Inport  Port=2
  Neural network output : MATLAB Function  TreatAsAtomicUnit=on
  Update of neural weight : MATLAB Function  TreatAsAtomicUnit=on
  Weight initialisation : MATLAB Function  TreatAsAtomicUnit=on
  Weight update : Integrator  InitialConditionSource=external
  w_i : Outport
  wires:
  Update of neural weight/1(W_dot) -> Weight update/1
  esti_s/1 -> Update of neural weight/2(esti_s)
  state/1 -> Update of neural weight/1(phi_net), Neural network output/1(phi_net)
  Neural network output/1(w_i) -> w_i/1
  Weight initialisation/1(W_0) -> Weight update/2
  Weight update/1 -> Update of neural weight/3(W), Neural network output/2(W)

== system Multi_drones_deri_compare/Controller 3/Controller/Attitude controller/Sliding mode differentiator/First-order derivative ==
  ang_d : Inport
  t : Inport  Port=2
  First derivative : MATLAB Function  TreatAsAtomicUnit=on
  Memory : Memory  InitialCondition=[0;0;0]
  Memory1 : Memory
  Memory2 : Memory  InitialCondition=[0;0;0]
  ang_d_dot : Outport
  wires:
  ang_d/1 -> First derivative/1(ang_d)
  First derivative/1(ang_d_dot) -> Memory2/1
  t/1 -> First derivative/2(t)
  First derivative/3(loop_num) -> Memory1/1
  Memory1/1 -> First derivative/5("loop_num ")
  First derivative/2(ang_d_prev) -> Memory/1
  Memory/1 -> First derivative/3("ang_d_prev ")
  Memory2/1 -> First derivative/4("ang_d_dot "), ang_d_dot/1

== system Multi_drones_deri_compare/Controller 3/Controller/Attitude controller/Sliding mode differentiator/Second-order derivative ==
  ang_d_dot : Inport
  t : Inport  Port=2
  First derivative : MATLAB Function  TreatAsAtomicUnit=on
  Memory : Memory  InitialCondition=[0;0;0]
  Memory1 : Memory
  Memory2 : Memory  InitialCondition=[0;0;0]
  ang_d_ddot : Outport
  wires:
  ang_d_dot/1 -> First derivative/1(ang_d_dot)
  First derivative/1(ang_d_ddot) -> Memory2/1
  t/1 -> First derivative/2(t)
  First derivative/3(loop_num) -> Memory1/1
  Memory1/1 -> First derivative/5("loop_num ")
  First derivative/2(ang_d_dot_prev) -> Memory/1
  Memory/1 -> First derivative/3("ang_d_dot_prev ")
  Memory2/1 -> First derivative/4("ang_d_ddot "), ang_d_ddot/1

== system Multi_drones_deri_compare/Controller 3/Controller/Position controller1/Position loop observer/Single Layer Neural network ==
  state : Inport
  esti_s : Inport  Port=2
  Neural network output : MATLAB Function  TreatAsAtomicUnit=on
  Update of neural weight : MATLAB Function  TreatAsAtomicUnit=on
  Weight initialisation : MATLAB Function  TreatAsAtomicUnit=on
  Weight update : Integrator  InitialConditionSource=external
  w_i : Outport
  wires:
  Update of neural weight/1(W_dot) -> Weight update/1
  esti_s/1 -> Update of neural weight/2(esti_s)
  state/1 -> Update of neural weight/1(phi_net), Neural network output/1(phi_net)
  Neural network output/1(w_i) -> w_i/1
  Weight initialisation/1(W_0) -> Weight update/2
  Weight update/1 -> Update of neural weight/3(W), Neural network output/2(W)

== system Multi_drones_deri_compare/Controller 4/Controller/Attitude controller/Attitude loop observer/Single Layer Neural network ==
  state : Inport
  esti_s : Inport  Port=2
  Neural network output : MATLAB Function  TreatAsAtomicUnit=on
  Update of neural weight : MATLAB Function  TreatAsAtomicUnit=on
  Weight initialisation : MATLAB Function  TreatAsAtomicUnit=on
  Weight update : Integrator  InitialConditionSource=external
  w_i : Outport
  wires:
  Update of neural weight/1(W_dot) -> Weight update/1
  esti_s/1 -> Update of neural weight/2(esti_s)
  state/1 -> Update of neural weight/1(phi_net), Neural network output/1(phi_net)
  Neural network output/1(w_i) -> w_i/1
  Weight initialisation/1(W_0) -> Weight update/2
  Weight update/1 -> Update of neural weight/3(W), Neural network output/2(W)

== system Multi_drones_deri_compare/Controller 4/Controller/Attitude controller/Sliding mode differentiator/First-order derivative ==
  ang_d : Inport
  t : Inport  Port=2
  First derivative : MATLAB Function  TreatAsAtomicUnit=on
  Memory : Memory  InitialCondition=[0;0;0]
  Memory1 : Memory
  Memory2 : Memory  InitialCondition=[0;0;0]
  ang_d_dot : Outport
  wires:
  ang_d/1 -> First derivative/1(ang_d)
  First derivative/1(ang_d_dot) -> Memory2/1
  t/1 -> First derivative/2(t)
  First derivative/3(loop_num) -> Memory1/1
  Memory1/1 -> First derivative/5("loop_num ")
  First derivative/2(ang_d_prev) -> Memory/1
  Memory/1 -> First derivative/3("ang_d_prev ")
  Memory2/1 -> First derivative/4("ang_d_dot "), ang_d_dot/1

== system Multi_drones_deri_compare/Controller 4/Controller/Attitude controller/Sliding mode differentiator/Second-order derivative ==
  ang_d_dot : Inport
  t : Inport  Port=2
  First derivative : MATLAB Function  TreatAsAtomicUnit=on
  Memory : Memory  InitialCondition=[0;0;0]
  Memory1 : Memory
  Memory2 : Memory  InitialCondition=[0;0;0]
  ang_d_ddot : Outport
  wires:
  ang_d_dot/1 -> First derivative/1(ang_d_dot)
  First derivative/1(ang_d_ddot) -> Memory2/1
  t/1 -> First derivative/2(t)
  First derivative/3(loop_num) -> Memory1/1
  Memory1/1 -> First derivative/5("loop_num ")
  First derivative/2(ang_d_dot_prev) -> Memory/1
  Memory/1 -> First derivative/3("ang_d_dot_prev ")
  Memory2/1 -> First derivative/4("ang_d_ddot "), ang_d_ddot/1
